simulink model "LargeSignalStablizerDesign"  (R2023a)
settings: Solver=VariableStepAuto  StartTime=0.0  StopTime=21  FixedStep=1e-6  RelTol=1e-3  EnableMultiTasking=on
InitFcn:
  | fswitch=25e3;
  | Ldc=2000e-6;
  | Cdc=470e-6;
  | E0=100;
  | Vref=170;
  | 
  | 
  | 
  | Ldc=2000e-6;
  | Cdc=470e-6;
  | Vdc_in1=100;
  | Vdc_out=170;
  | D1=Vdc_in1/Vdc_out;
  | inta=0.35;
  | wi1=(1/15)*fswitch*2*pi;
  | kbat_cp=(1/sqrt(inta^2+1))*wi1*Ldc/Vdc_out;
  | kbat_ci=inta*wi1*kbat_cp;
  | wv1=(1/12)*wi1;
  | kbat_vp=(1/sqrt(inta^2+1))*wv1*Cdc/D1;
  | kbat_vi=inta*wv1*kbat_vp;
libraries: spsControlledVoltageSourceLib x4, spsCurrentMeasurementLib x4, slpidlib x4, spsControlledCurrentSourceLib x2, spsVoltageMeasurementLib x2, spsSeriesRLCBranchLib x2, spsStairGeneratorLib x2, spspowerguiLib x1
settings Model: Creator=pengf  LastModifiedBy=pengf
settings SolverCC: AlgebraicLoopSolver=TrustRegion
settings DataIOCC: LimitDataPoints=on  SaveFormat=Array  ReturnWorkspaceOutputs=off
settings OptimizationCC: LifeSpan=inf
settings DebuggingCC: ParameterPrecisionLossMsg=none  UnconnectedInputMsg=warning  UnconnectedOutputMsg=warning  UnconnectedLineMsg=warning  AllowSymbolicDim=off  SFUnexpectedBacktrackingDiag=warning  SFNoUnconditionalDefaultTransitionDiag=warning  SFExecutionAtInitializationDiag=none  ArithmeticOperatorsInVariantConditions=warning
settings HardwareCC: ProdBitPerPointer=32  ProdBitPerSizeT=32  ProdBitPerPtrDiffT=32  ProdLargestAtomicFloat=None  ProdIntDivRoundTo=Undefined  ProdEndianess=Unspecified  ProdWordSize=32  ProdHWDeviceType=32-bit Generic
settings ModelReferenceCC: EnableRefExpFcnMdlSchedulingChecks=on  PropagateSignalLabelsOutOfModel=off
settings SFSimCC: SimUseLocalCustomCode=off  CustomCodeUndefinedFunction=UseInterfaceOnly
settings RTWCC: RTWUseLocalCustomCode=off
settings CodeAppCC: StateflowObjectComments=on
settings GRTTargetCC: TargetLangStandard=C89/C90 (ANSI)
settings ConfigComp: CovMetricSettings=dw  CovSaveCumulativeToWorkspaceVar=on  CovSaveSingleToWorkspaceVar=on  CovExternalEMLEnable=off
settings SimscapeCC: SimscapeNormalizeSystem=off

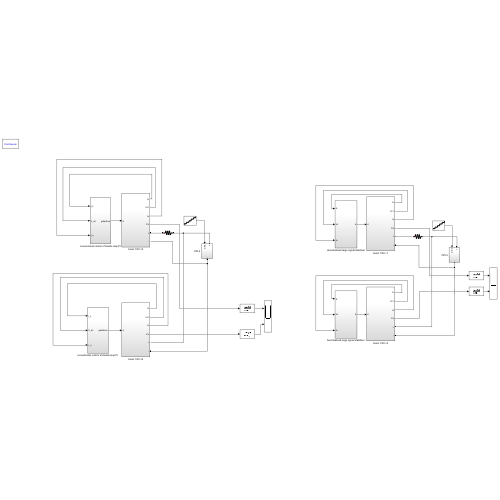
[thumbnail: Simulink's stored preview of the top-level diagram]
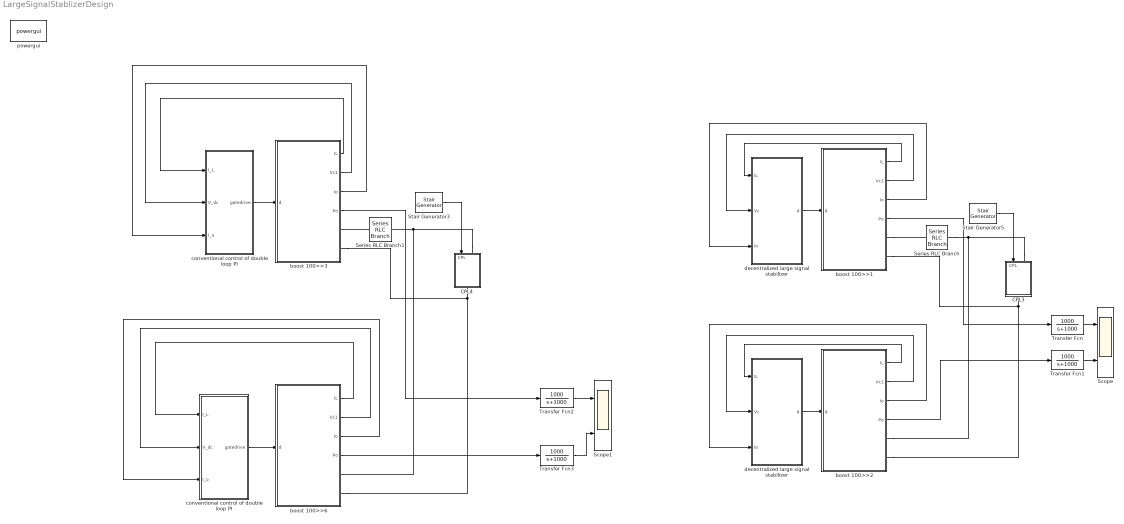
== system LargeSignalStablizerDesign ==
  CPL3 : Subsystem
  CPL4 : Subsystem
  Scope : Scope  NumInputPorts=2
  Scope1 : Scope  NumInputPorts=2
  Series RLC Branch : spsSeriesRLCBranchLib/Series RLC Branch  LConnTagsString=__new0  RConnTagsString=__new0  BranchType=R  Resistance=0.1  Inductance=1e-3  SetiL0=off  InitialCurrent=0  Capacitance=1e-6  Setx0=off  InitialVoltage=0  Measurements=None
  Series RLC Branch1 : spsSeriesRLCBranchLib/Series RLC Branch  LConnTagsString=__new0  RConnTagsString=__new0  BranchType=R  Resistance=0.1  Inductance=1e-3  SetiL0=off  InitialCurrent=0  Capacitance=1e-6  Setx0=off  InitialVoltage=0  Measurements=None
  Stair Generator3 : spsStairGeneratorLib/Stair Generator  t=[0, 3 6 9 12 15 18]  e="[0 500 1000  1500 2000 2500 3000]"  Ts=0
  Stair Generator5 : spsStairGeneratorLib/Stair Generator  t=[0, 3 6 9 12 15 18]  e="[0 500 1000  1500 2000 2500 3000]"  Ts=0
  Transfer Fcn{,1..3} (4 alike) : TransferFcn  Numerator=[1000]  Denominator=[1 1000]
  boost 100>>1 : Subsystem
  boost 100>>2 : Subsystem
  boost 100>>3 : Subsystem
  boost 100>>6 : Subsystem
  conventional control of double loop PI : Subsystem
  "conventional control of double loop PI " : Subsystem
  decentralized large signal stabilizer : Subsystem
  "decentralized large signal stabilizer " : Subsystem
  powergui : spspowerguiLib/powergui  Priority=1  SimulationMode=Continuous  SampleTime=1e-6  frequency=60  Iterations=50  frequencyindice=0  Pbase=100e6  ErrMax=1e-4  UnitsV=kV  UnitsW=MW  buscounter=0  FunctionMessages=off  echomessages=off  EnableUseOfTLC=off  CurrentSourceSwitches=off  DisableSnubberDevices=off  DisableRonSwitches=off  DisableVfSwitches=off  DisplayEquations=off  AutomaticDiscreteSolvers=off  SolverType=Tustin/Backward Euler (TBE)  Interpol=off  ExternalGateDelay=off  methode=off  Ts=100  x0status=blocks  SPID=off  SwTol=0  HookPort=off  NonlinearTolerance=1e-4  nMaxIteration=100  ContinueOnMaxIteration=off  RestoreLinks=warning  ResistiveCurrentMeasurement=off  Frange=[0:2:500]  Ylog=off  Xlog=on  ShowGrid=off  save=off  variable=ZData  structure=ScopeData1  ZoomFFT=off  StartTime=0.1  cycles=30  DisplayStyle=3  fundamental=1  FreqAxis=off  MaxFrequency=1000  frequencyindicesteady=1  RmsSteady=1  display=off
  wires:
  boost 100>>1/2(Vc1) -> decentralized large signal stabilizer/2(Vc)
  decentralized large signal stabilizer/1(d) -> boost 100>>1/1(d)
  boost 100>>1/3(Io) -> decentralized large signal stabilizer/3(Io)
  boost 100>>1/1(IL) -> decentralized large signal stabilizer/1(IL)
  Stair Generator5/1 -> CPL3/1(CPL)
  boost 100>>2/2(Vc1) -> "decentralized large signal stabilizer "/2(Vc)
  "decentralized large signal stabilizer "/1(d) -> boost 100>>2/1(d)
  boost 100>>2/3(Io) -> "decentralized large signal stabilizer "/3(Io)
  boost 100>>2/1(IL) -> "decentralized large signal stabilizer "/1(IL)
  boost 100>>1/4(Po) -> Transfer Fcn/1
  boost 100>>2/4(Po) -> Transfer Fcn1/1
  conventional control of double loop PI/1(gatedrive) -> boost 100>>3/1(d)
  Stair Generator3/1 -> CPL4/1(CPL)
  boost 100>>3/1(IL) -> conventional control of double loop PI/1(I_L)
  boost 100>>3/2(Vc1) -> conventional control of double loop PI/2(V_dc)
  Transfer Fcn/1 -> Scope/1
  Transfer Fcn1/1 -> Scope/2
  "conventional control of double loop PI "/1(gatedrive) -> boost 100>>6/1(d)
  boost 100>>6/1(IL) -> "conventional control of double loop PI "/1(I_L)
  boost 100>>6/2(Vc1) -> "conventional control of double loop PI "/2(V_dc)
  boost 100>>3/3(Io) -> conventional control of double loop PI/3(I_o)
  boost 100>>6/3(Io) -> "conventional control of double loop PI "/3(I_o)
  boost 100>>3/4(Po) -> Transfer Fcn2/1
  boost 100>>6/4(Po) -> Transfer Fcn3/1
  Transfer Fcn3/1 -> Scope1/2
  Transfer Fcn2/1 -> Scope1/1
  connections:
  boost 100>>1/RConn2 -- CPL3/RConn1 -- boost 100>>2/RConn2
  boost 100>>1/RConn1 -- Series RLC Branch/LConn1
  boost 100>>3/RConn2 -- CPL4/RConn1 -- boost 100>>6/RConn2
  CPL3/LConn1 -- boost 100>>2/RConn1 -- Series RLC Branch/RConn1
  CPL4/LConn1 -- boost 100>>6/RConn1 -- Series RLC Branch1/RConn1
  Series RLC Branch1/LConn1 -- boost 100>>3/RConn1

== system LargeSignalStablizerDesign/CPL3 ==
  CPL : Inport
  Controlled Current Source1 : spsControlledCurrentSourceLib/Controlled Current Source  Initialize=on  Source_Type=AC  Amplitude=0  Phase=0  Frequency=0  Measurements=None
  Divide : Product  Inputs=*/
  Saturation : Saturate  UpperLimit=inf  LowerLimit=0.1
  Voltage Measurement : spsVoltageMeasurementLib/Voltage Measurement  PhasorSimulation=off  OutputType=Complex  PSBequivalent=0
  + : PMIOPort  Side=Left
  - : PMIOPort  Port=2  Side=Right
  wires:
  CPL/1 -> Divide/1
  Saturation/1 -> Divide/2
  Divide/1 -> Controlled Current Source1/1
  Voltage Measurement/1 -> Saturation/1
  connections:
  Voltage Measurement/LConn2 -- Controlled Current Source1/RConn1 -- -/RConn1
  Voltage Measurement/LConn1 -- +/RConn1 -- Controlled Current Source1/LConn1

== system LargeSignalStablizerDesign/CPL4 ==
  CPL : Inport
  Controlled Current Source1 : spsControlledCurrentSourceLib/Controlled Current Source  Initialize=on  Source_Type=AC  Amplitude=0  Phase=0  Frequency=0  Measurements=None
  Divide : Product  Inputs=*/
  Saturation : Saturate  UpperLimit=inf  LowerLimit=0.1
  Voltage Measurement : spsVoltageMeasurementLib/Voltage Measurement  PhasorSimulation=off  OutputType=Complex  PSBequivalent=0
  + : PMIOPort  Side=Left
  - : PMIOPort  Port=2  Side=Right
  wires:
  Voltage Measurement/1 -> Saturation/1
  Divide/1 -> Controlled Current Source1/1
  Saturation/1 -> Divide/2
  CPL/1 -> Divide/1
  connections:
  Controlled Current Source1/LConn1 -- +/RConn1 -- Voltage Measurement/LConn1
  -/RConn1 -- Controlled Current Source1/RConn1 -- Voltage Measurement/LConn2

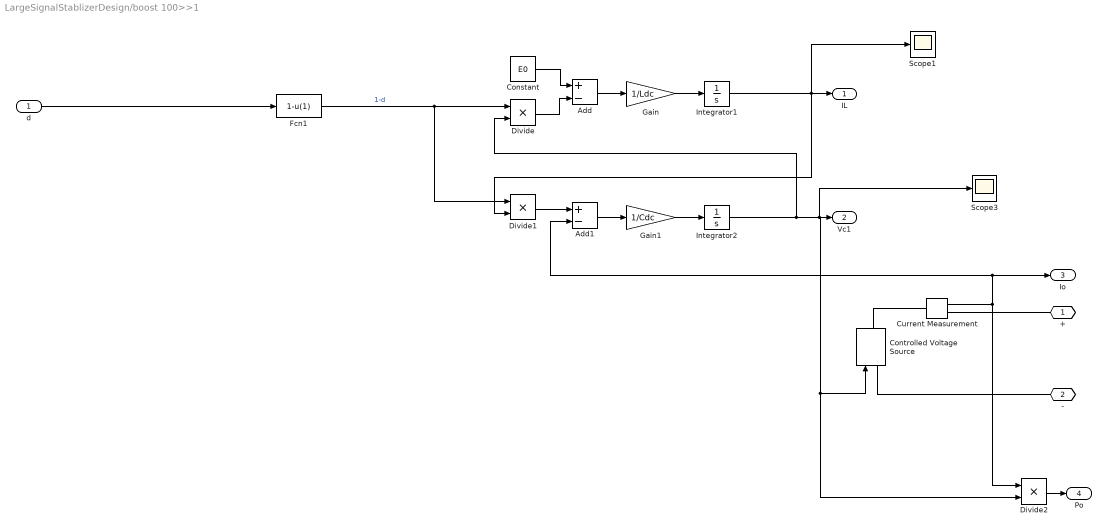
== system LargeSignalStablizerDesign/boost 100>>1 ==
  d : Inport
  Add : Sum  Inputs=+-
  Add1 : Sum  Inputs=+-
  Constant : Constant  Value=E0
  Controlled Voltage Source : spsControlledVoltageSourceLib/Controlled Voltage Source  Initialize=on  Source_Type=AC  Amplitude=0  Phase=0  Frequency=0  Measurements=None
  Current Measurement : spsCurrentMeasurementLib/Current Measurement  PhasorSimulation=off  OutputType=Complex  PSBequivalent=0
  Divide : Product  Inputs=**
  Divide1 : Product  Inputs=**
  Divide2 : Product  Inputs=**
  Fcn1 : Fcn  Expr=1-u(1)
  Gain : Gain  Gain=1/Ldc
  Gain1 : Gain  Gain=1/Cdc
  Integrator1 : Integrator
  Integrator2 : Integrator  InitialCondition=Vref
  Scope1 : Scope
  Scope3 : Scope
  + : PMIOPort  Side=Right
  - : PMIOPort  Port=2  Side=Right
  IL : Outport
  Vc1 : Outport  Port=2
  Io : Outport  Port=3
  Po : Outport  Port=4
  wires:
  Divide2/1 -> Po/1
  Gain/1 -> Integrator1/1
  Add/1 -> Gain/1
  Constant/1 -> Add/1
  Divide/1 -> Add/2
  Gain1/1 -> Integrator2/1
  Add1/1 -> Gain1/1
  Divide1/1 -> Add1/1
  Integrator1/1 -> IL/1, Scope1/1, Divide1/2
  Integrator2/1 -> Scope3/1, Controlled Voltage Source/1, Divide2/2, Vc1/1, Divide/2
  Fcn1/1 -> Divide1/1, Divide/1  "1-d"
  Current Measurement/1 -> Divide2/1, Io/1, Add1/2
  d/1 -> Fcn1/1
  connections:
  Current Measurement/RConn1 -- +/RConn1
  Controlled Voltage Source/LConn1 -- -/RConn1
  Current Measurement/LConn1 -- Controlled Voltage Source/RConn1

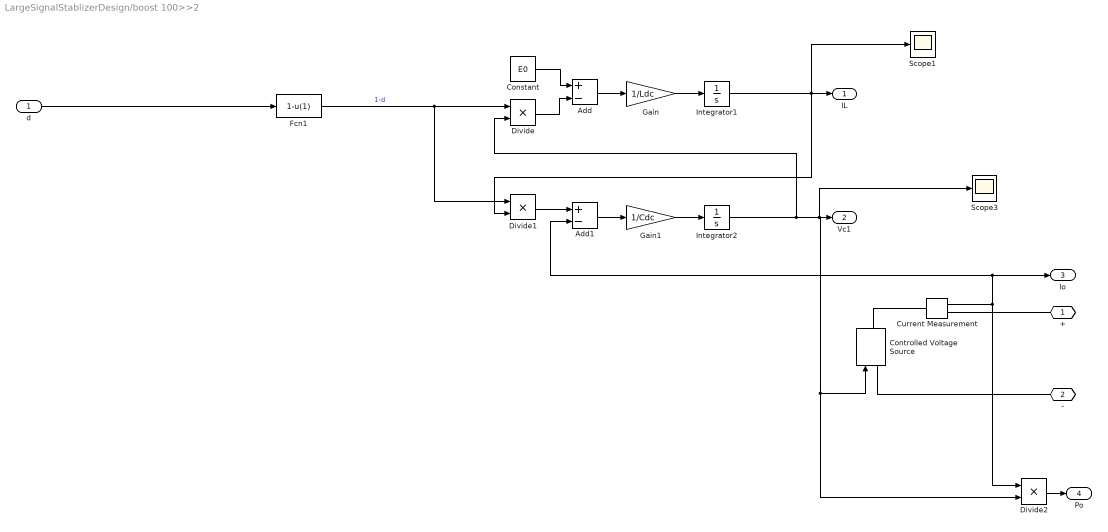
== system LargeSignalStablizerDesign/boost 100>>2 ==
  d : Inport
  Add : Sum  Inputs=+-
  Add1 : Sum  Inputs=+-
  Constant : Constant  Value=E0
  Controlled Voltage Source : spsControlledVoltageSourceLib/Controlled Voltage Source  Initialize=on  Source_Type=AC  Amplitude=0  Phase=0  Frequency=0  Measurements=None
  Current Measurement : spsCurrentMeasurementLib/Current Measurement  PhasorSimulation=off  OutputType=Complex  PSBequivalent=0
  Divide : Product  Inputs=**
  Divide1 : Product  Inputs=**
  Divide2 : Product  Inputs=**
  Fcn1 : Fcn  Expr=1-u(1)
  Gain : Gain  Gain=1/Ldc
  Gain1 : Gain  Gain=1/Cdc
  Integrator1 : Integrator
  Integrator2 : Integrator  InitialCondition=Vref
  Scope1 : Scope
  Scope3 : Scope
  + : PMIOPort  Side=Right
  - : PMIOPort  Port=2  Side=Right
  IL : Outport
  Vc1 : Outport  Port=2
  Io : Outport  Port=3
  Po : Outport  Port=4
  wires:
  d/1 -> Fcn1/1
  Current Measurement/1 -> Add1/2, Io/1, Divide2/1
  Fcn1/1 -> Divide/1, Divide1/1  "1-d"
  Integrator2/1 -> Divide/2, Vc1/1, Divide2/2, Controlled Voltage Source/1, Scope3/1
  Integrator1/1 -> Divide1/2, Scope1/1, IL/1
  Divide1/1 -> Add1/1
  Add1/1 -> Gain1/1
  Gain1/1 -> Integrator2/1
  Divide/1 -> Add/2
  Constant/1 -> Add/1
  Add/1 -> Gain/1
  Gain/1 -> Integrator1/1
  Divide2/1 -> Po/1
  connections:
  Current Measurement/LConn1 -- Controlled Voltage Source/RConn1
  Controlled Voltage Source/LConn1 -- -/RConn1
  Current Measurement/RConn1 -- +/RConn1

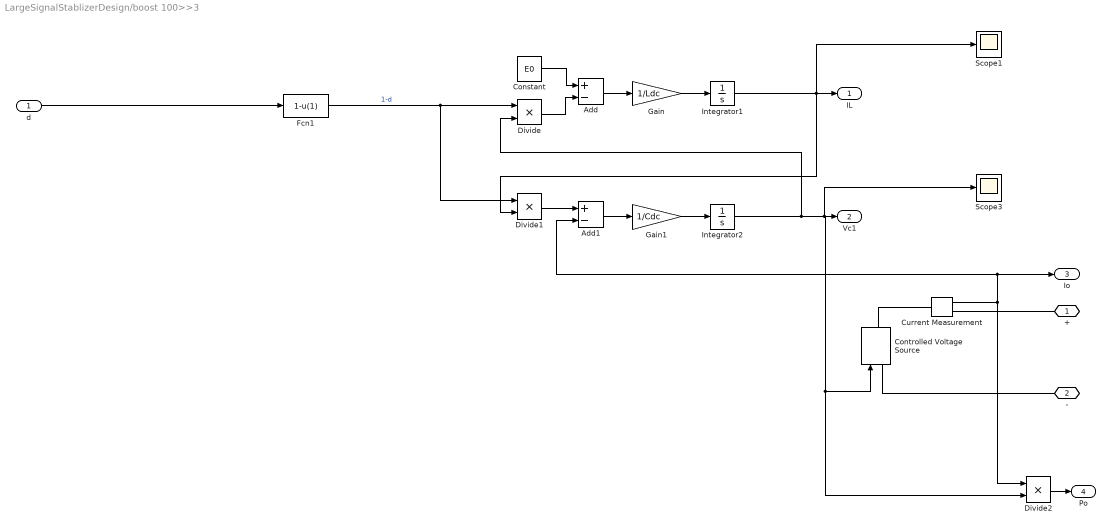
== system LargeSignalStablizerDesign/boost 100>>3 ==
  d : Inport
  Add : Sum  Inputs=+-
  Add1 : Sum  Inputs=+-
  Constant : Constant  Value=E0
  Controlled Voltage Source : spsControlledVoltageSourceLib/Controlled Voltage Source  Initialize=on  Source_Type=AC  Amplitude=0  Phase=0  Frequency=0  Measurements=None
  Current Measurement : spsCurrentMeasurementLib/Current Measurement  PhasorSimulation=off  OutputType=Complex  PSBequivalent=0
  Divide : Product  Inputs=**
  Divide1 : Product  Inputs=**
  Divide2 : Product  Inputs=**
  Fcn1 : Fcn  Expr=1-u(1)
  Gain : Gain  Gain=1/Ldc
  Gain1 : Gain  Gain=1/Cdc
  Integrator1 : Integrator
  Integrator2 : Integrator  InitialCondition=Vref
  Scope1 : Scope
  Scope3 : Scope
  + : PMIOPort  Side=Right
  - : PMIOPort  Port=2  Side=Right
  IL : Outport
  Vc1 : Outport  Port=2
  Io : Outport  Port=3
  Po : Outport  Port=4
  wires:
  d/1 -> Fcn1/1
  Current Measurement/1 -> Add1/2, Io/1, Divide2/1
  Fcn1/1 -> Divide/1, Divide1/1  "1-d"
  Integrator2/1 -> Divide/2, Vc1/1, Divide2/2, Controlled Voltage Source/1, Scope3/1
  Integrator1/1 -> IL/1, Divide1/2, Scope1/1
  Divide1/1 -> Add1/1
  Add1/1 -> Gain1/1
  Gain1/1 -> Integrator2/1
  Divide/1 -> Add/2
  Constant/1 -> Add/1
  Add/1 -> Gain/1
  Gain/1 -> Integrator1/1
  Divide2/1 -> Po/1
  connections:
  Current Measurement/LConn1 -- Controlled Voltage Source/RConn1
  Controlled Voltage Source/LConn1 -- -/RConn1
  Current Measurement/RConn1 -- +/RConn1

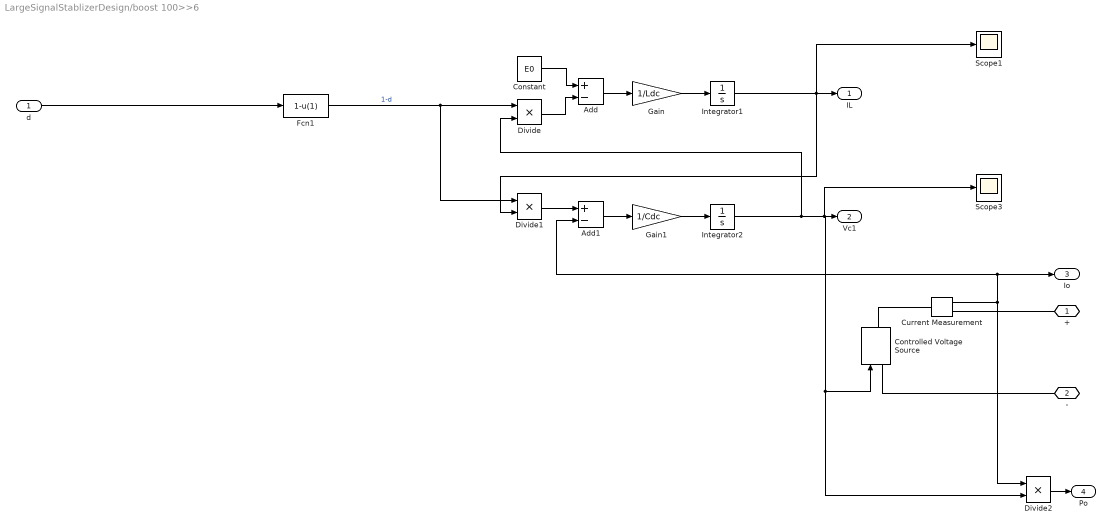
== system LargeSignalStablizerDesign/boost 100>>6 ==
  d : Inport
  Add : Sum  Inputs=+-
  Add1 : Sum  Inputs=+-
  Constant : Constant  Value=E0
  Controlled Voltage Source : spsControlledVoltageSourceLib/Controlled Voltage Source  Initialize=on  Source_Type=AC  Amplitude=0  Phase=0  Frequency=0  Measurements=None
  Current Measurement : spsCurrentMeasurementLib/Current Measurement  PhasorSimulation=off  OutputType=Complex  PSBequivalent=0
  Divide : Product  Inputs=**
  Divide1 : Product  Inputs=**
  Divide2 : Product  Inputs=**
  Fcn1 : Fcn  Expr=1-u(1)
  Gain : Gain  Gain=1/Ldc
  Gain1 : Gain  Gain=1/Cdc
  Integrator1 : Integrator
  Integrator2 : Integrator  InitialCondition=Vref
  Scope1 : Scope
  Scope3 : Scope
  + : PMIOPort  Side=Right
  - : PMIOPort  Port=2  Side=Right
  IL : Outport
  Vc1 : Outport  Port=2
  Io : Outport  Port=3
  Po : Outport  Port=4
  wires:
  Divide2/1 -> Po/1
  Gain/1 -> Integrator1/1
  Add/1 -> Gain/1
  Constant/1 -> Add/1
  Divide/1 -> Add/2
  Gain1/1 -> Integrator2/1
  Add1/1 -> Gain1/1
  Divide1/1 -> Add1/1
  Integrator1/1 -> Scope1/1, Divide1/2, IL/1
  Integrator2/1 -> Scope3/1, Controlled Voltage Source/1, Divide2/2, Vc1/1, Divide/2
  Fcn1/1 -> Divide1/1, Divide/1  "1-d"
  Current Measurement/1 -> Divide2/1, Io/1, Add1/2
  d/1 -> Fcn1/1
  connections:
  Current Measurement/RConn1 -- +/RConn1
  Controlled Voltage Source/LConn1 -- -/RConn1
  Current Measurement/LConn1 -- Controlled Voltage Source/RConn1

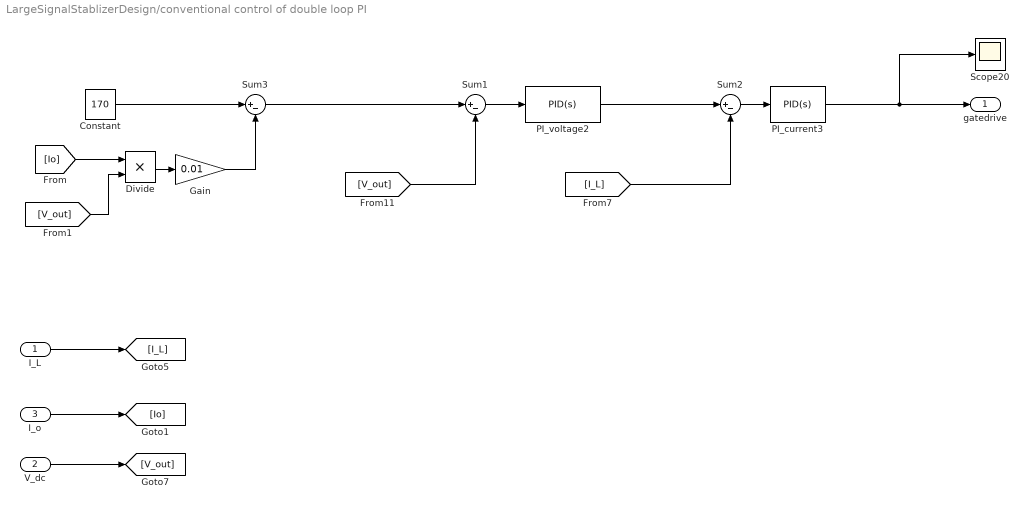
== system LargeSignalStablizerDesign/conventional control of double loop PI ==
  I_L : Inport
  V_dc : Inport  Port=2
  I_o : Inport  Port=3
  Constant : Constant  Value=170
  Divide : Product  Inputs=**
  Gain : Gain  Gain=0.01
  PI_current3 : slpidlib/PID Controller  Controller=PID  Form=Parallel  TimeDomain=Continuous-time  UseExternalTs=off  SampleTime=-1  IntegratorMethod=Forward Euler  FilterMethod=Forward Euler  ControllerParametersSource=internal  P=kbat_cp  I=kbat_ci  UseKiTs=off  D=0  N=100  UseFilter=on  TunerSelectOption=Transfer Function Based (PID Tuner App)  InitialConditionSource=internal  InitialConditionForIntegrator=0  InitialConditionForFilter=0  DifferentiatorICPrevScaledInput=0  ExternalReset=none  TrackingMode=off  Kt=1  LimitOutput=on  SatLimitsSource=internal  UpperSaturationLimit=0.99  LowerSaturationLimit=0.01  LinearizeAsGain=on  AntiWindupMode=none  Kb=1  LimitIntegrator=off  UpperIntegratorSaturationLimit=inf  LowerIntegratorSaturationLimit=-inf  POutMin=[]  POutMax=[]  IOutMin=[]  IOutMax=[]  DOutMin=[]  DOutMax=[]  NOutMin=[]  NOutMax=[]  SumOutMin=[]  SumOutMax=[]  SaturationOutMin=[]  SaturationOutMax=[]  PParamMin=[]  PParamMax=[]  IParamMin=[]  IParamMax=[]  DParamMin=[]  DParamMax=[]  NParamMin=[]  NParamMax=[]  KbParamMin=[]  KbParamMax=[]  KtParamMin=[]  KtParamMax=[]  KbOutMin=[]  KbOutMax=[]  KtOutMin=[]  KtOutMax=[]  IntegratorOutMin=[]  IntegratorOutMax=[]  FilterOutMin=[]  FilterOutMax=[]  SumI1OutMin=[]  SumI1OutMax=[]  SumI2OutMin=[]  SumI2OutMax=[]  SumI3OutMin=[]  SumI3OutMax=[]  SumI4OutMin=[]  SumI4OutMax=[]  SumDOutMin=[]  SumDOutMax=[]  DifferentiatorOutMin=[]  DifferentiatorOutMax=[]  FilterDiffOutCoefMin=[]  FilterDiffOutCoefMax=[]  ReciprocalOutMin=[]  ReciprocalOutMax=[]  SumDenOutMin=[]  SumDenOutMax=[]  SumNumOutMin=[]  SumNumOutMax=[]  DivideOutMin=[]  DivideOutMax=[]  UdiffTsProdOutMin=[]  UdiffTsProdOutMax=[]  NTsProdOutMin=[]  NTsProdOutMax=[]  UintegralTsProdOutMin=[]  UintegralTsProdOutMax=[]  UngainTsProdOutMin=[]  UngainTsProdOutMax=[]  ClampingZeroOutDataTypeStr=Inherit: Inherit via back propagation  ClampingZeroOutMin=[]  ClampingZeroOutMax=[]  FilterDenConstantOutDataTypeStr=Inherit: Inherit via back propagation  FilterDenConstantOutMin=[]  FilterDenConstantOutMax=[]  PCopyOutDataTypeStr=Inherit: Inherit via back propagation  PCopyOutMin=[]  PCopyOutMax=[]  NCopyOutDataTypeStr=Inherit: Inherit via back propagation  NCopyOutMin=[]  NCopyOutMax=[]  IntegratorContinuousStateAttributes=''  IntegratorStateMustResolveToSignalObject=off  IntegratorRTWStateStorageClass=Auto  FilterContinuousStateAttributes=''  FilterStateMustResolveToSignalObject=off  FilterRTWStateStorageClass=Auto  ParallelPVariant=InternalParameters  IdealPVariant=Disabled  IVariant=InternalParameters  DVariant=InternalParameters  IntegratorVariant=Continuous  SatVariant=Disabled  AWVariant=Passthrough  PCopyVariant=Disabled  TRVariant=Disabled  FdbkBlocksVariant=Forward  IdealPFdbkVariant=Disabled  SatFdbkVariant=Disabled  DerivativeFilterVariant=ContFilter  NVariant=InternalParameters  NCopyVariant=Disabled  FilterICVariant=InternalICsFilter  IntegratorICVariant=InternalICs  ExternalResetVariant=Disabled  TRSumVariant=Passthrough  SumFdbkVariant=Disabled  SumVariant=Sum_PID  TsampFilterVariant=InternalTs  TsampNgainVariant=Passthrough  TsampIntegralVariant=Passthrough  ExternalSaturationOutDataTypeStr=Inherit: Same as second input
  PI_voltage2 : slpidlib/PID Controller  Controller=PID  Form=Parallel  TimeDomain=Continuous-time  UseExternalTs=off  SampleTime=-1  IntegratorMethod=Forward Euler  FilterMethod=Forward Euler  ControllerParametersSource=internal  P=kbat_vp  I=kbat_vi  UseKiTs=off  D=0  N=100  UseFilter=on  TunerSelectOption=Transfer Function Based (PID Tuner App)  InitialConditionSource=internal  InitialConditionForIntegrator=0  InitialConditionForFilter=0  DifferentiatorICPrevScaledInput=0  ExternalReset=none  TrackingMode=off  Kt=1  LimitOutput=on  SatLimitsSource=internal  UpperSaturationLimit=150  LowerSaturationLimit=-150  LinearizeAsGain=on  AntiWindupMode=none  Kb=1  LimitIntegrator=off  UpperIntegratorSaturationLimit=inf  LowerIntegratorSaturationLimit=-inf  POutMin=[]  POutMax=[]  IOutMin=[]  IOutMax=[]  DOutMin=[]  DOutMax=[]  NOutMin=[]  NOutMax=[]  SumOutMin=[]  SumOutMax=[]  SaturationOutMin=[]  SaturationOutMax=[]  PParamMin=[]  PParamMax=[]  IParamMin=[]  IParamMax=[]  DParamMin=[]  DParamMax=[]  NParamMin=[]  NParamMax=[]  KbParamMin=[]  KbParamMax=[]  KtParamMin=[]  KtParamMax=[]  KbOutMin=[]  KbOutMax=[]  KtOutMin=[]  KtOutMax=[]  IntegratorOutMin=[]  IntegratorOutMax=[]  FilterOutMin=[]  FilterOutMax=[]  SumI1OutMin=[]  SumI1OutMax=[]  SumI2OutMin=[]  SumI2OutMax=[]  SumI3OutMin=[]  SumI3OutMax=[]  SumI4OutMin=[]  SumI4OutMax=[]  SumDOutMin=[]  SumDOutMax=[]  DifferentiatorOutMin=[]  DifferentiatorOutMax=[]  FilterDiffOutCoefMin=[]  FilterDiffOutCoefMax=[]  ReciprocalOutMin=[]  ReciprocalOutMax=[]  SumDenOutMin=[]  SumDenOutMax=[]  SumNumOutMin=[]  SumNumOutMax=[]  DivideOutMin=[]  DivideOutMax=[]  UdiffTsProdOutMin=[]  UdiffTsProdOutMax=[]  NTsProdOutMin=[]  NTsProdOutMax=[]  UintegralTsProdOutMin=[]  UintegralTsProdOutMax=[]  UngainTsProdOutMin=[]  UngainTsProdOutMax=[]  ClampingZeroOutDataTypeStr=Inherit: Inherit via back propagation  ClampingZeroOutMin=[]  ClampingZeroOutMax=[]  FilterDenConstantOutDataTypeStr=Inherit: Inherit via back propagation  FilterDenConstantOutMin=[]  FilterDenConstantOutMax=[]  PCopyOutDataTypeStr=Inherit: Inherit via back propagation  PCopyOutMin=[]  PCopyOutMax=[]  NCopyOutDataTypeStr=Inherit: Inherit via back propagation  NCopyOutMin=[]  NCopyOutMax=[]  IntegratorContinuousStateAttributes=''  IntegratorStateMustResolveToSignalObject=off  IntegratorRTWStateStorageClass=Auto  FilterContinuousStateAttributes=''  FilterStateMustResolveToSignalObject=off  FilterRTWStateStorageClass=Auto  ParallelPVariant=InternalParameters  IdealPVariant=Disabled  IVariant=InternalParameters  DVariant=InternalParameters  IntegratorVariant=Continuous  SatVariant=Enabled  AWVariant=Passthrough  PCopyVariant=Disabled  TRVariant=Disabled  FdbkBlocksVariant=Forward  IdealPFdbkVariant=Disabled  SatFdbkVariant=Disabled  DerivativeFilterVariant=ContFilter  NVariant=InternalParameters  NCopyVariant=Disabled  FilterICVariant=InternalICsFilter  IntegratorICVariant=InternalICs  ExternalResetVariant=Disabled  TRSumVariant=Passthrough  SumFdbkVariant=Disabled  SumVariant=Sum_PID  TsampFilterVariant=InternalTs  TsampNgainVariant=Passthrough  TsampIntegralVariant=Disabled_SignalSpec  ExternalSaturationOutDataTypeStr=Inherit: Same as second input
  Scope20 : Scope
  Sum1 : Sum  Inputs=|+-
  Sum2 : Sum  Inputs=|+-
  Sum3 : Sum  Inputs=|+-
  gatedrive : Outport
  wires:
  V_dc/1 -> [V_out]
  I_L/1 -> [I_L]
  [V_out] -> Sum1/2
  PI_voltage2/1 -> Sum2/1
  Sum1/1 -> PI_voltage2/1
  [I_L] -> Sum2/2
  Sum2/1 -> PI_current3/1
  PI_current3/1 -> gatedrive/1, Scope20/1
  I_o/1 -> [Io]
  [Io] -> Divide/1
  [V_out] -> Divide/2
  Divide/1 -> Gain/1
  Sum3/1 -> Sum1/1
  Constant/1 -> Sum3/1
  Gain/1 -> Sum3/2

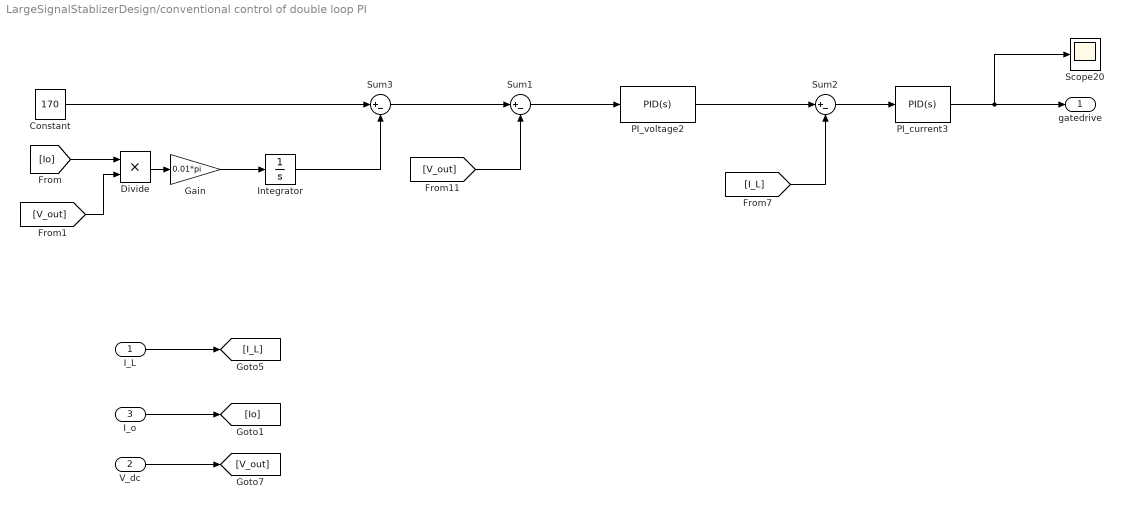
== system LargeSignalStablizerDesign/conventional control of double loop PI  ==
  I_L : Inport
  V_dc : Inport  Port=2
  I_o : Inport  Port=3
  Constant : Constant  Value=170
  Divide : Product  Inputs=**
  Gain : Gain  Gain=0.01*pi
  Integrator : Integrator
  PI_current3 : slpidlib/PID Controller  Controller=PID  Form=Parallel  TimeDomain=Continuous-time  UseExternalTs=off  SampleTime=-1  IntegratorMethod=Forward Euler  FilterMethod=Forward Euler  ControllerParametersSource=internal  P=kbat_cp  I=kbat_ci  UseKiTs=off  D=0  N=100  UseFilter=on  TunerSelectOption=Transfer Function Based (PID Tuner App)  InitialConditionSource=internal  InitialConditionForIntegrator=0  InitialConditionForFilter=0  DifferentiatorICPrevScaledInput=0  ExternalReset=none  TrackingMode=off  Kt=1  LimitOutput=on  SatLimitsSource=internal  UpperSaturationLimit=0.99  LowerSaturationLimit=0.01  LinearizeAsGain=on  AntiWindupMode=none  Kb=1  LimitIntegrator=off  UpperIntegratorSaturationLimit=inf  LowerIntegratorSaturationLimit=-inf  POutMin=[]  POutMax=[]  IOutMin=[]  IOutMax=[]  DOutMin=[]  DOutMax=[]  NOutMin=[]  NOutMax=[]  SumOutMin=[]  SumOutMax=[]  SaturationOutMin=[]  SaturationOutMax=[]  PParamMin=[]  PParamMax=[]  IParamMin=[]  IParamMax=[]  DParamMin=[]  DParamMax=[]  NParamMin=[]  NParamMax=[]  KbParamMin=[]  KbParamMax=[]  KtParamMin=[]  KtParamMax=[]  KbOutMin=[]  KbOutMax=[]  KtOutMin=[]  KtOutMax=[]  IntegratorOutMin=[]  IntegratorOutMax=[]  FilterOutMin=[]  FilterOutMax=[]  SumI1OutMin=[]  SumI1OutMax=[]  SumI2OutMin=[]  SumI2OutMax=[]  SumI3OutMin=[]  SumI3OutMax=[]  SumI4OutMin=[]  SumI4OutMax=[]  SumDOutMin=[]  SumDOutMax=[]  DifferentiatorOutMin=[]  DifferentiatorOutMax=[]  FilterDiffOutCoefMin=[]  FilterDiffOutCoefMax=[]  ReciprocalOutMin=[]  ReciprocalOutMax=[]  SumDenOutMin=[]  SumDenOutMax=[]  SumNumOutMin=[]  SumNumOutMax=[]  DivideOutMin=[]  DivideOutMax=[]  UdiffTsProdOutMin=[]  UdiffTsProdOutMax=[]  NTsProdOutMin=[]  NTsProdOutMax=[]  UintegralTsProdOutMin=[]  UintegralTsProdOutMax=[]  UngainTsProdOutMin=[]  UngainTsProdOutMax=[]  ClampingZeroOutDataTypeStr=Inherit: Inherit via back propagation  ClampingZeroOutMin=[]  ClampingZeroOutMax=[]  FilterDenConstantOutDataTypeStr=Inherit: Inherit via back propagation  FilterDenConstantOutMin=[]  FilterDenConstantOutMax=[]  PCopyOutDataTypeStr=Inherit: Inherit via back propagation  PCopyOutMin=[]  PCopyOutMax=[]  NCopyOutDataTypeStr=Inherit: Inherit via back propagation  NCopyOutMin=[]  NCopyOutMax=[]  IntegratorContinuousStateAttributes=''  IntegratorStateMustResolveToSignalObject=off  IntegratorRTWStateStorageClass=Auto  FilterContinuousStateAttributes=''  FilterStateMustResolveToSignalObject=off  FilterRTWStateStorageClass=Auto  ParallelPVariant=InternalParameters  IdealPVariant=Disabled  IVariant=InternalParameters  DVariant=InternalParameters  IntegratorVariant=Continuous  SatVariant=Disabled  AWVariant=Passthrough  PCopyVariant=Disabled  TRVariant=Disabled  FdbkBlocksVariant=Forward  IdealPFdbkVariant=Disabled  SatFdbkVariant=Disabled  DerivativeFilterVariant=ContFilter  NVariant=InternalParameters  NCopyVariant=Disabled  FilterICVariant=InternalICsFilter  IntegratorICVariant=InternalICs  ExternalResetVariant=Disabled  TRSumVariant=Passthrough  SumFdbkVariant=Disabled  SumVariant=Sum_PID  TsampFilterVariant=InternalTs  TsampNgainVariant=Passthrough  TsampIntegralVariant=Passthrough  ExternalSaturationOutDataTypeStr=Inherit: Same as second input
  PI_voltage2 : slpidlib/PID Controller  Controller=PID  Form=Parallel  TimeDomain=Continuous-time  UseExternalTs=off  SampleTime=-1  IntegratorMethod=Forward Euler  FilterMethod=Forward Euler  ControllerParametersSource=internal  P=kbat_vp  I=kbat_vi  UseKiTs=off  D=0  N=100  UseFilter=on  TunerSelectOption=Transfer Function Based (PID Tuner App)  InitialConditionSource=internal  InitialConditionForIntegrator=0  InitialConditionForFilter=0  DifferentiatorICPrevScaledInput=0  ExternalReset=none  TrackingMode=off  Kt=1  LimitOutput=on  SatLimitsSource=internal  UpperSaturationLimit=150  LowerSaturationLimit=-150  LinearizeAsGain=on  AntiWindupMode=none  Kb=1  LimitIntegrator=off  UpperIntegratorSaturationLimit=inf  LowerIntegratorSaturationLimit=-inf  POutMin=[]  POutMax=[]  IOutMin=[]  IOutMax=[]  DOutMin=[]  DOutMax=[]  NOutMin=[]  NOutMax=[]  SumOutMin=[]  SumOutMax=[]  SaturationOutMin=[]  SaturationOutMax=[]  PParamMin=[]  PParamMax=[]  IParamMin=[]  IParamMax=[]  DParamMin=[]  DParamMax=[]  NParamMin=[]  NParamMax=[]  KbParamMin=[]  KbParamMax=[]  KtParamMin=[]  KtParamMax=[]  KbOutMin=[]  KbOutMax=[]  KtOutMin=[]  KtOutMax=[]  IntegratorOutMin=[]  IntegratorOutMax=[]  FilterOutMin=[]  FilterOutMax=[]  SumI1OutMin=[]  SumI1OutMax=[]  SumI2OutMin=[]  SumI2OutMax=[]  SumI3OutMin=[]  SumI3OutMax=[]  SumI4OutMin=[]  SumI4OutMax=[]  SumDOutMin=[]  SumDOutMax=[]  DifferentiatorOutMin=[]  DifferentiatorOutMax=[]  FilterDiffOutCoefMin=[]  FilterDiffOutCoefMax=[]  ReciprocalOutMin=[]  ReciprocalOutMax=[]  SumDenOutMin=[]  SumDenOutMax=[]  SumNumOutMin=[]  SumNumOutMax=[]  DivideOutMin=[]  DivideOutMax=[]  UdiffTsProdOutMin=[]  UdiffTsProdOutMax=[]  NTsProdOutMin=[]  NTsProdOutMax=[]  UintegralTsProdOutMin=[]  UintegralTsProdOutMax=[]  UngainTsProdOutMin=[]  UngainTsProdOutMax=[]  ClampingZeroOutDataTypeStr=Inherit: Inherit via back propagation  ClampingZeroOutMin=[]  ClampingZeroOutMax=[]  FilterDenConstantOutDataTypeStr=Inherit: Inherit via back propagation  FilterDenConstantOutMin=[]  FilterDenConstantOutMax=[]  PCopyOutDataTypeStr=Inherit: Inherit via back propagation  PCopyOutMin=[]  PCopyOutMax=[]  NCopyOutDataTypeStr=Inherit: Inherit via back propagation  NCopyOutMin=[]  NCopyOutMax=[]  IntegratorContinuousStateAttributes=''  IntegratorStateMustResolveToSignalObject=off  IntegratorRTWStateStorageClass=Auto  FilterContinuousStateAttributes=''  FilterStateMustResolveToSignalObject=off  FilterRTWStateStorageClass=Auto  ParallelPVariant=InternalParameters  IdealPVariant=Disabled  IVariant=InternalParameters  DVariant=InternalParameters  IntegratorVariant=Continuous  SatVariant=Enabled  AWVariant=Passthrough  PCopyVariant=Disabled  TRVariant=Disabled  FdbkBlocksVariant=Forward  IdealPFdbkVariant=Disabled  SatFdbkVariant=Disabled  DerivativeFilterVariant=ContFilter  NVariant=InternalParameters  NCopyVariant=Disabled  FilterICVariant=InternalICsFilter  IntegratorICVariant=InternalICs  ExternalResetVariant=Disabled  TRSumVariant=Passthrough  SumFdbkVariant=Disabled  SumVariant=Sum_PID  TsampFilterVariant=InternalTs  TsampNgainVariant=Passthrough  TsampIntegralVariant=Disabled_SignalSpec  ExternalSaturationOutDataTypeStr=Inherit: Same as second input
  Scope20 : Scope
  Sum1 : Sum  Inputs=|+-
  Sum2 : Sum  Inputs=|+-
  Sum3 : Sum  Inputs=|+-
  gatedrive : Outport
  wires:
  Gain/1 -> Integrator/1
  Constant/1 -> Sum3/1
  Sum3/1 -> Sum1/1
  Divide/1 -> Gain/1
  [V_out] -> Divide/2
  [Io] -> Divide/1
  I_o/1 -> [Io]
  PI_current3/1 -> Scope20/1, gatedrive/1
  Sum2/1 -> PI_current3/1
  [I_L] -> Sum2/2
  Sum1/1 -> PI_voltage2/1
  PI_voltage2/1 -> Sum2/1
  [V_out] -> Sum1/2
  I_L/1 -> [I_L]
  V_dc/1 -> [V_out]
  Integrator/1 -> Sum3/2

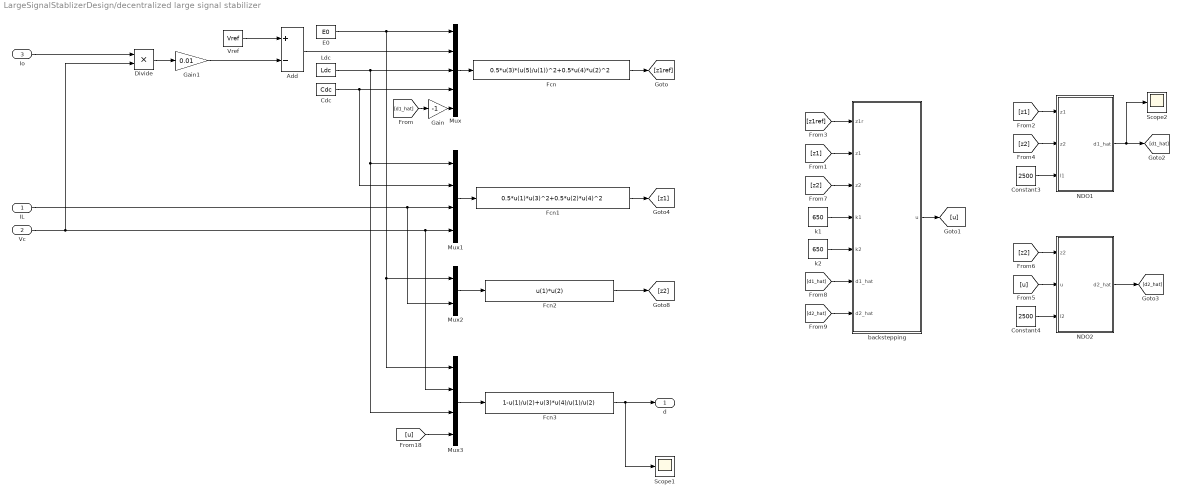
== system LargeSignalStablizerDesign/decentralized large signal stabilizer ==
  IL : Inport
  Vc : Inport  Port=2
  Io : Inport  Port=3
  Add : Sum  Inputs=+-
  Cdc : Constant  Value=Cdc
  Constant3 : Constant  Value=2500
  Constant4 : Constant  Value=2500
  Divide : Product  Inputs=**
  E0 : Constant  Value=E0
  Fcn : Fcn  Expr=0.5*u(3)*(u(5)/u(1))^2+0.5*u(4)*u(2)^2
  Fcn1 : Fcn  Expr=0.5*u(1)*u(3)^2+0.5*u(2)*u(4)^2
  Fcn2 : Fcn  Expr=u(1)*u(2)
  Fcn3 : Fcn  Expr=1-u(1)/u(2)+u(3)*u(4)/u(1)/u(2)
  Gain : Gain  Gain=-1
  Gain1 : Gain  Gain=0.01
  Ldc : Constant  Value=Ldc
  Mux : Mux  Inputs=5
  Mux1 : Mux
  Mux2 : Mux  Inputs=2
  Mux3 : Mux
  NDO1 : Subsystem
  NDO2 : Subsystem
  Scope1 : Scope
  Scope2 : Scope
  "Vref " : Constant  Value=Vref
  backstepping : MATLAB Function  TreatAsAtomicUnit=on
  k1 : Constant  Value=650
  k2 : Constant  Value=650
  d : Outport
  wires:
  Add/1 -> Mux/2
  [d1_hat] -> Gain/1
  Gain/1 -> Mux/5
  E0/1 -> Mux3/1, Mux2/1, Mux/1
  Ldc/1 -> Mux1/1, Mux3/3, Mux/3
  Cdc/1 -> Mux1/2, Mux/4
  Fcn2/1 -> [z2]
  Fcn1/1 -> [z1]
  IL/1 -> Mux2/2, Mux1/3
  Mux1/1 -> Fcn1/1
  Mux3/1 -> Fcn3/1
  Mux2/1 -> Fcn2/1
  [u] -> Mux3/4
  Mux/1 -> Fcn/1
  Fcn/1 -> [z1ref]
  Vc/1 -> Divide/2, Mux3/2, Mux1/4
  "Vref "/1 -> Add/1
  Fcn3/1 -> d/1, Scope1/1
  Io/1 -> Divide/1
  Divide/1 -> Gain1/1
  [z1] -> NDO1/1(z1)
  [z2] -> NDO1/2(z2)
  NDO1/1(d1_hat) -> Scope2/1, [d1_hat]
  Constant3/1 -> NDO1/3(l1)
  NDO2/1(d2_hat) -> [d2_hat]
  Constant4/1 -> NDO2/3(l2)
  [z2] -> NDO2/1(z2)
  k1/1 -> backstepping/4(k1)
  k2/1 -> backstepping/5(k2)
  [z1ref] -> backstepping/1(z1r)
  [z1] -> backstepping/2(z1)
  [z2] -> backstepping/3(z2)
  [d1_hat] -> backstepping/6(d1_hat)
  [d2_hat] -> backstepping/7(d2_hat)
  backstepping/1(u) -> [u]
  [u] -> NDO2/2(u)
  Gain1/1 -> Add/2

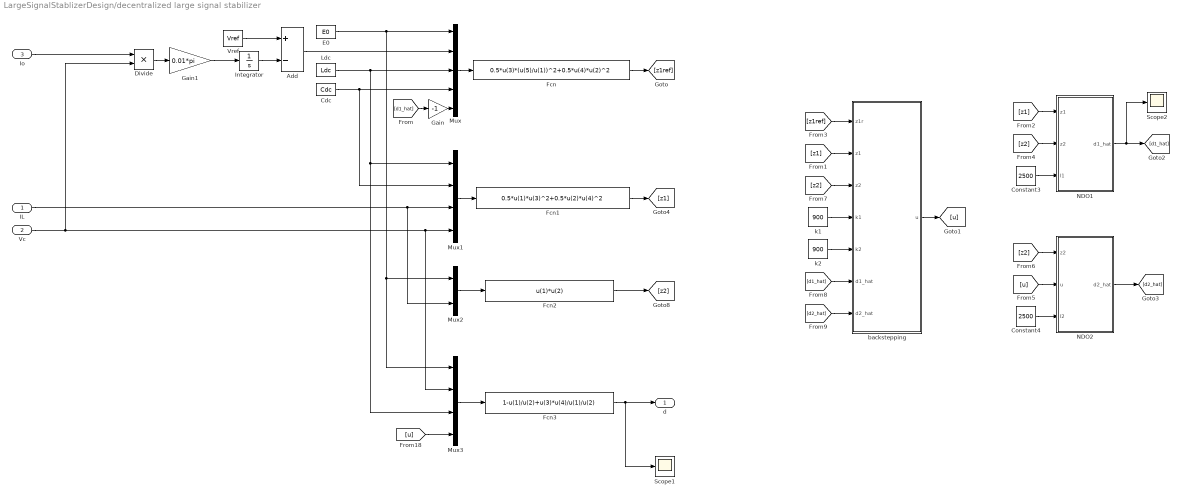
== system LargeSignalStablizerDesign/decentralized large signal stabilizer  ==
  IL : Inport
  Vc : Inport  Port=2
  Io : Inport  Port=3
  Add : Sum  Inputs=+-
  Cdc : Constant  Value=Cdc
  Constant3 : Constant  Value=2500
  Constant4 : Constant  Value=2500
  Divide : Product  Inputs=**
  E0 : Constant  Value=E0
  Fcn : Fcn  Expr=0.5*u(3)*(u(5)/u(1))^2+0.5*u(4)*u(2)^2
  Fcn1 : Fcn  Expr=0.5*u(1)*u(3)^2+0.5*u(2)*u(4)^2
  Fcn2 : Fcn  Expr=u(1)*u(2)
  Fcn3 : Fcn  Expr=1-u(1)/u(2)+u(3)*u(4)/u(1)/u(2)
  Gain : Gain  Gain=-1
  Gain1 : Gain  Gain=0.01*pi
  Integrator : Integrator
  Ldc : Constant  Value=Ldc
  Mux : Mux  Inputs=5
  Mux1 : Mux
  Mux2 : Mux  Inputs=2
  Mux3 : Mux
  NDO1 : Subsystem
  NDO2 : Subsystem
  Scope1 : Scope
  Scope2 : Scope
  "Vref " : Constant  Value=Vref
  backstepping : MATLAB Function  TreatAsAtomicUnit=on
  k1 : Constant  Value=900
  k2 : Constant  Value=900
  d : Outport
  wires:
  [u] -> NDO2/2(u)
  backstepping/1(u) -> [u]
  [d2_hat] -> backstepping/7(d2_hat)
  [d1_hat] -> backstepping/6(d1_hat)
  [z2] -> backstepping/3(z2)
  [z1] -> backstepping/2(z1)
  [z1ref] -> backstepping/1(z1r)
  k2/1 -> backstepping/5(k2)
  k1/1 -> backstepping/4(k1)
  [z2] -> NDO2/1(z2)
  Constant4/1 -> NDO2/3(l2)
  NDO2/1(d2_hat) -> [d2_hat]
  Constant3/1 -> NDO1/3(l1)
  NDO1/1(d1_hat) -> [d1_hat], Scope2/1
  [z2] -> NDO1/2(z2)
  [z1] -> NDO1/1(z1)
  Divide/1 -> Gain1/1
  Io/1 -> Divide/1
  Fcn3/1 -> Scope1/1, d/1
  "Vref "/1 -> Add/1
  Vc/1 -> Mux1/4, Mux3/2, Divide/2
  Fcn/1 -> [z1ref]
  Mux/1 -> Fcn/1
  [u] -> Mux3/4
  Mux2/1 -> Fcn2/1
  Mux3/1 -> Fcn3/1
  Mux1/1 -> Fcn1/1
  IL/1 -> Mux1/3, Mux2/2
  Fcn1/1 -> [z1]
  Fcn2/1 -> [z2]
  Cdc/1 -> Mux/4, Mux1/2
  Ldc/1 -> Mux/3, Mux3/3, Mux1/1
  E0/1 -> Mux/1, Mux2/1, Mux3/1
  Gain/1 -> Mux/5
  [d1_hat] -> Gain/1
  Add/1 -> Mux/2
  Gain1/1 -> Integrator/1
  Integrator/1 -> Add/2

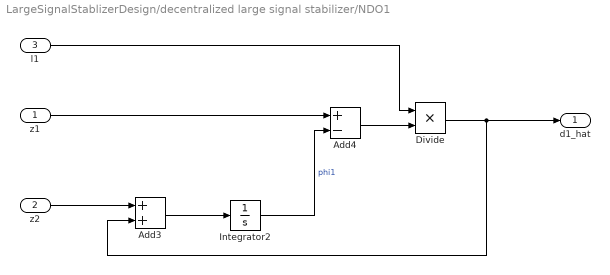
== system LargeSignalStablizerDesign/decentralized large signal stabilizer/NDO1 ==
  z1 : Inport
  z2 : Inport  Port=2
  l1 : Inport  Port=3
  Add3 : Sum
  Add4 : Sum  Inputs=+-
  Divide : Product  Inputs=**
  Integrator2 : Integrator
  d1_hat : Outport
  wires:
  l1/1 -> Divide/1
  z1/1 -> Add4/1
  z2/1 -> Add3/1
  Add3/1 -> Integrator2/1
  Add4/1 -> Divide/2
  Divide/1 -> d1_hat/1, Add3/2
  Integrator2/1 -> Add4/2  "phi1"

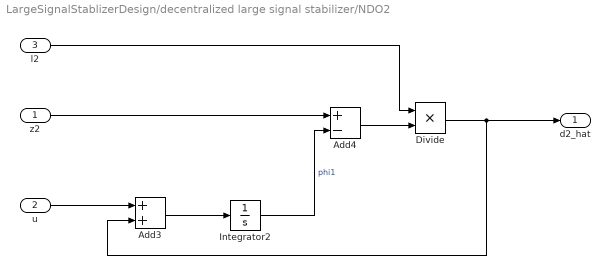
== system LargeSignalStablizerDesign/decentralized large signal stabilizer/NDO2 ==
  z2 : Inport
  u : Inport  Port=2
  l2 : Inport  Port=3
  Add3 : Sum
  Add4 : Sum  Inputs=+-
  Divide : Product  Inputs=**
  Integrator2 : Integrator
  d2_hat : Outport
  wires:
  Integrator2/1 -> Add4/2  "phi1"
  Divide/1 -> Add3/2, d2_hat/1
  Add4/1 -> Divide/2
  Add3/1 -> Integrator2/1
  u/1 -> Add3/1
  z2/1 -> Add4/1
  l2/1 -> Divide/1

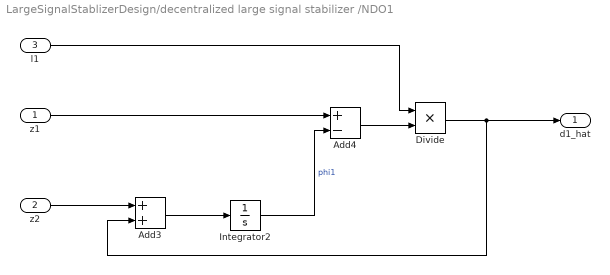
== system LargeSignalStablizerDesign/decentralized large signal stabilizer /NDO1 ==
  z1 : Inport
  z2 : Inport  Port=2
  l1 : Inport  Port=3
  Add3 : Sum
  Add4 : Sum  Inputs=+-
  Divide : Product  Inputs=**
  Integrator2 : Integrator
  d1_hat : Outport
  wires:
  Integrator2/1 -> Add4/2  "phi1"
  Divide/1 -> Add3/2, d1_hat/1
  Add4/1 -> Divide/2
  Add3/1 -> Integrator2/1
  z2/1 -> Add3/1
  z1/1 -> Add4/1
  l1/1 -> Divide/1

== system LargeSignalStablizerDesign/decentralized large signal stabilizer /NDO2 ==
  z2 : Inport
  u : Inport  Port=2
  l2 : Inport  Port=3
  Add3 : Sum
  Add4 : Sum  Inputs=+-
  Divide : Product  Inputs=**
  Integrator2 : Integrator
  d2_hat : Outport
  wires:
  l2/1 -> Divide/1
  z2/1 -> Add4/1
  u/1 -> Add3/1
  Add3/1 -> Integrator2/1
  Add4/1 -> Divide/2
  Divide/1 -> d2_hat/1, Add3/2
  Integrator2/1 -> Add4/2  "phi1"

== matlab function LargeSignalStablizerDesign/decentralized large signal stabilizer/backstepping ==
  data: z1r input; u output; z1 input; z2 input; k1 input; k2 input; d1_hat input; d2_hat input
function u = fcn(z1r,z1,z2,k1,k2,d1_hat,d2_hat)
e1=z1-z1r;
z2r=-k1*e1-d1_hat;
e2=z2-z2r;
u=-k2*e2-d2_hat-k1*(z2+d1_hat);

== matlab function LargeSignalStablizerDesign/decentralized large signal stabilizer /backstepping ==
  data: z1r input; u output; z1 input; z2 input; k1 input; k2 input; d1_hat input; d2_hat input
function u = fcn(z1r,z1,z2,k1,k2,d1_hat,d2_hat)
e1=z1-z1r;
z2r=-k1*e1-d1_hat;
e2=z2-z2r;
u=-k2*e2-d2_hat-k1*(z2+d1_hat);
